simulink model "flexcan_and_fm_over_can_s32k14x"  (Simulink 9.0)
settings: Solver=FixedStepDiscrete  StartTime=0.0  StopTime=10.0  FixedStep=0.1  RelTol=1e-3  EnableMultiTasking=on
InitFcn:
  | mbd_s32k_consistency_checks(bdroot(gcs));
undefined symbols (not defined in the file): LQFP
libraries: mbd_s32k1xx_ec_toolbox x9, simulink x1
Description:
  | This model tests freemaster over CAN0 interface and use CAN1 interface to communicate
  | with other device (eg.: S32K118EVB).
  | 
  | 
  | Validation:
  | 
  | Build flexcan_loopback32k11x.mdl project on S32k118 EVB
  | Build flexcan_and_fm_over_can_s32k14x.mdl on S32k144 EVB
  | Make sure you connect S32K144 through CAN1 interface to S32k118
  | 
  | Open "flexcan_and_fm_over_can_s32k14x.pmp" freemaster project, connect to S32K144
  | board through CAN0 interface at 1Mbps and modify 'CAN_send' variable from Freemaster to '1'.
  | 
  | Once the 'CAN_send' variable is set to 1, a numeric sequence with ID 0x3FF is send once on FlexCAN1 at 500Kbps, Red LED will light
  | for a short period. The S32K144 board will listen for
  | a message with ID 0x3FE over the same CAN1 and once it was received, the 'CAN_send' variable will be cleared.
  | 
  | - The CAN0 (Freemaster) Baudrate is set to 1Mbps and CAN1 Baudrate is set to 500Kbps.
  | -S32K118EVB-Q064 (or any other device who can receive a message over can interface and send back a message with
  | ID 0x3FE)
  | 
  | HW prerequisite:
  | - S32K144EVB-Q100
  | - S32K118EVB-Q064 (or any other device who can receive a message over can interface and send back a message with
  | ID 0x3FE)
  | 
  | - Make sure that external power supply is provided through J16.
settings Model: Creator=agrigorev  LastModifiedBy=nxf35172
settings DataIOCC: ExternalInput=off  InitialState=off  LimitDataPoints=on  SaveOutput=off  SignalLogging=off  SaveTime=off
settings OptimizationCC: DefaultParameterBehavior=Inlined  LifeSpan=1
settings DebuggingCC: SolverPrmCheckMsg=warning  InheritedTsInSrcMsg=none  SingleTaskRateTransMsg=error  UnconnectedInputMsg=error  UnconnectedOutputMsg=error  UnconnectedLineMsg=error  AllowSymbolicDim=off  UnknownTsInhSupMsg=error  StateNameClashWarn=warning
settings HardwareCC: ProdLargestAtomicInteger=Long  ProdLargestAtomicFloat=Double  ProdIntDivRoundTo=Zero  ProdEndianess=LittleEndian  ProdHWDeviceType=ARM Compatible->ARM Cortex
settings SFSimCC: MATLABDynamicMemAlloc=off
settings RTWCC: SystemTargetFile=mbd_s32k.tlc  MakeCommand=mbd_s32k_make_rtw COPY_MDLREF_INCLUDES=0  TemplateMakefile=mbd_s32k.tmf  Description=Model Based Design Toolbox S32K14x Code Generation Target  GenerateReport=on  IncludeHyperlinkInReport=on  LaunchReport=on  GenerateTraceInfo=on  GenerateTraceReport=on  GenerateTraceReportSl=on  GenerateTraceReportSf=on  GenerateTraceReportEml=on
settings CodeAppCC: ForceParamTrailComments=on  IgnoreCustomStorageClasses=off  OperatorAnnotations=on  SimulinkDataObjDesc=on  SFDataObjDesc=on  MATLABFcnDesc=on  InsertBlockDesc=on  MATLABSourceComments=on
settings STFCustomTargetCC: CombineOutputUpdateFcns=on  ERTCustomFileBanners=on  SupportContinuousTime=off  SupportNonInlinedSFcns=off  RemoveResetFunc=on  MATLABClassNameForMDSCustomization=Simulink.SoftwareTarget.ERTCustomization  GRTInterface=off  SystemTargetFile=mbd_s32k14.tlc
settings ERTTargetCC: MultiwordLength=2048  ParMdlRefBuildCompliant=off  CompOptLevelCompliant=off  ConcurrentExecutionCompliant=off  ModelStepFunctionPrototypeControlCompliant=off  CPPClassGenCompliant=off  UseToolchainInfoCompliant=off  InlinedParameterPlacement=NonHierarchical  ERTSrcFileBannerTemplate=mbd_ert_code_template.cgt  ERTHdrFileBannerTemplate=mbd_ert_code_template.cgt  ERTDataSrcFileTemplate=mbd_ert_code_template.cgt  ERTDataHdrFileTemplate=mbd_ert_code_template.cgt  ERTCustomFileTemplate=example_file_process.tlc

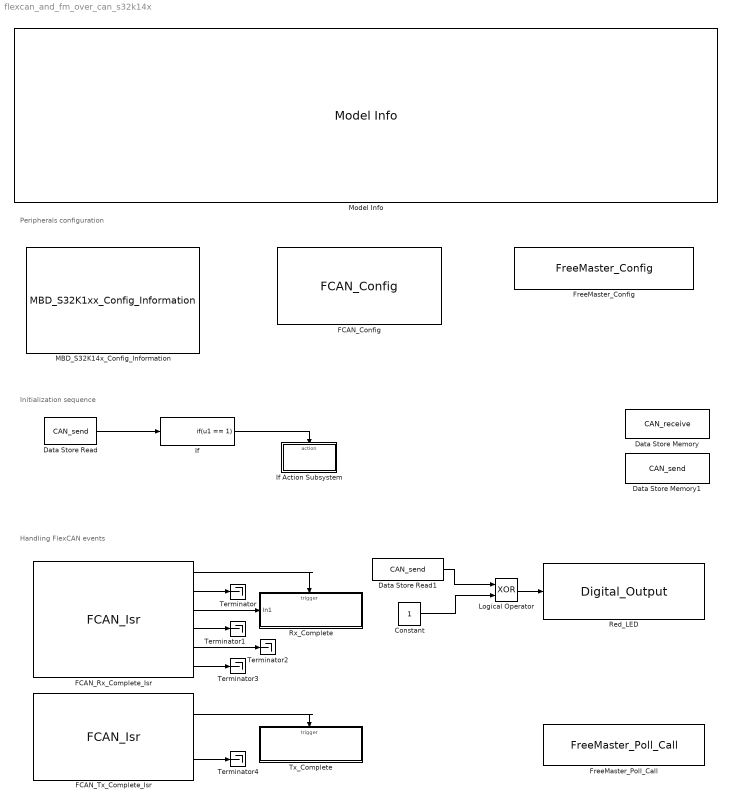
== system flexcan_and_fm_over_can_s32k14x ==
  note: Peripherals configuration
  note: Handling FlexCAN events
  note: Initialization sequence
  Constant : Constant  OutDataTypeStr=boolean
  Data Store Memory : DataStoreMemory  DataStoreName=CAN_receive  ReadBeforeWriteMsg=warning  WriteAfterWriteMsg=warning  WriteAfterReadMsg=warning  ShowAdditionalParam=off  OutDataTypeStr=uint8
  Data Store Memory1 : DataStoreMemory  DataStoreName=CAN_send  ReadBeforeWriteMsg=warning  WriteAfterWriteMsg=warning  WriteAfterReadMsg=warning  ShowAdditionalParam=off  OutDataTypeStr=boolean
  Data Store Read : DataStoreRead  DataStoreName=CAN_send
  Data Store Read1 : DataStoreRead  DataStoreName=CAN_send
  FCAN_Config : mbd_s32k1xx_ec_toolbox/Communication Blocks/CAN Blocks/FCAN_Config  Priority=1  can_instance=1  can_mode=Normal mode  can_max_num_mb=16  can_rx=PTA12: [CAN1_RX | CAN Rx channel]  can_tx=PTA13: [CAN1_TX | CAN Tx Channel]  show_adv_opts=on  can_clk_src=Peripheral clock  bitrate=500  bitrate_adv_opts=off  can_presdiv=7  can_rjw=3  can_pseg1=6  can_pseg2=3  can_propseg=7  can_cbt_presdiv=9  can_cbt_rjw=0  can_cbt_pseg1=3  can_cbt_pseg2=3  can_cbt_propseg=6  can_fd_enable=off  can_payload=8  can_rxfifo_enable=off  can_fifo_id_filter_extended=off  can_fifo_id_filter_remote=off  can_num_id_filters=8  can_fifo_id_format=A  can_fifo_id_filter={'0x0', '0x0', '0x0', '0x0', '0x0', '0x0', '0x0', '0x0'}  can_pn_enable=off  can_wakeup_match=off  can_wakeup_timeout=off  can_timeout_en=off  can_match_timeout=1  can_multiple_matches_en=off  can_num_matches=1  can_idfilter_extendedid=off  can_idfilter_remoteframe=off  can_idfilter_type=Match exact  can_idfilter_id1=0  can_idfilter_id2=0  can_payloadfilter_enable=on  can_payloadfilter_dlclow=0  can_payloadfilter_dlchigh=0  can_payloadfilter_type=Match exact  can_payloadfilter_payload1_b0=0  can_payloadfilter_payload1_b1=0  can_payloadfilter_payload1_b2=0  can_payloadfilter_payload1_b3=0  can_payloadfilter_payload1_b4=0  can_payloadfilter_payload1_b5=0  can_payloadfilter_payload1_b6=0  can_payloadfilter_payload1_b7=0  can_payloadfilter_payload2_b0=0  can_payloadfilter_payload2_b1=0  can_payloadfilter_payload2_b2=0  can_payloadfilter_payload2_b3=0  can_payloadfilter_payload2_b4=0  can_payloadfilter_payload2_b5=0  can_payloadfilter_payload2_b6=0  can_payloadfilter_payload2_b7=0
  FCAN_Rx_Complete_Isr : mbd_s32k1xx_ec_toolbox/Communication Blocks/CAN Blocks/FCAN_Isr  can_instance=1  can_event=Rx Complete
  FCAN_Tx_Complete_Isr : mbd_s32k1xx_ec_toolbox/Communication Blocks/CAN Blocks/FCAN_Isr  can_instance=1  can_event=Tx Complete
  FreeMaster_Config : mbd_s32k1xx_ec_toolbox/Utility Blocks/FreeMaster_Config  interface=CAN0  baudrate=1M  rxd=PTE4: [CAN0_RX | CAN Rx channel]  txd=PTE5: [CAN0_TX | CAN Tx Channel]  mode=Short Interrupt  isr_prio=0  show_adv_opts=on  use_scope=on  max_scope_vars=8  use_recorder=on  max_rec_vars=8  rec_buff_size=512  rec_timebase=10 milliseconds  comm_buffer_size_auto=on  comm_buffer_size=255  comm_rqueue_size_default=on  comm_rqueue_size=32
  FreeMaster_Poll_Call : mbd_s32k1xx_ec_toolbox/Utility Blocks/FreeMaster_Poll_Call
  If : If  IfExpression=u1 == 1  ShowElse=off
  If Action Subsystem : Subsystem  TreatAsAtomicUnit=on
  Logical Operator : Logic  Operator=XOR  AllPortsSameDT=off  OutDataTypeStr=boolean
  MBD_S32K14x_Config_Information : mbd_s32k1xx_ec_toolbox/MBD_S32K1xx_Config_Information  mbdt_ver=0  disp_str=|  config_params=[]  mcu_target_name=S32K144  mcu_target_package=100-LQFP  mcu_target_sram_size=48KB  mcu_system_clock_freq=80  mcu_xtal_freq=External 8  mcu_steptick_timer=LPIT Channel 0  mcu_steptick_prio=15  ds_import_enable=on  target_compiler=GCC  target_memory=FLASH  gcc_target_compile_opts=-mcpu=cortex-m4 -mthumb -mfloat-abi=hard -mfpu=fpv4-sp-d16 -O1 -g -gstrict-dwarf  gcc_target_assemble_opts=-mcpu=cortex-m4 -mthumb -mfloat-abi=hard -mfpu=fpv4-sp-d16 -g  gcc_target_link_opts=-mcpu=cortex-m4 -mthumb -mfloat-abi=hard -mfpu=fpv4-sp-d16  gcc_target_default_lcf=on  gcc_target_user_lcf=S32K144_48_flash.ld  ghs_target_compile_opts=-cpu=cortexm4f -thumb -DARM_MATH_CM4 -fpu=vfpv4_d16 -fsingle -Ogeneral -Wundef -Wimplicit-int -Wshadow -Wtrigraphs --no_commons --gnu_asm -gnu99 -gdwarf-2 -G  ghs_target_assemble_opts=-cpu=cortexm4f -fpu=vfpv4_d16  ghs_target_link_opts=-cpu=cortexm4f -thumb -fpu=vfpv4_d16  ghs_target_default_lcf=on  ghs_target_user_lcf=S32K144_48_flash.ld  iar_target_compile_opts=--cpu=Cortex-M4F --thumb --fpu=VFPv4_sp -Ol -e --debug --dlib_config normal  iar_target_assemble_opts=--cpu Cortex-M4F --thumb --fpu VFPv4_sp  iar_target_link_opts=--no_exceptions --vfe --inline  iar_target_default_lcf=on  iar_target_user_lcf=S32K144_48_flash.icf  pil_download_enable=off  rbl_download_enable=on  rbl_start_delay=5000000  rbl_download_interface=OpenSDA  rbl_restart_request=off  rbl_com_port=Custom  rbl_com_port_custom=COM1  pil_download_rate=57600  pil_opensda_drive=Custom  pil_opensda_drive_custom=D  pil_uart_instance=0  pil_uart_rx=PTA2: [LPUART0_RX | Receive]  pil_uart_tx=PTA3: [LPUART0_TX | Transmit]  FTM_PWM_PcrCheckEnDis=on  FTM_Input_Edge_Inputs_PcrCheckEnDis=on  FTM_Dual_Edge_Inputs_PcrCheckEnDis=on  FTM_Quadrature_Inputs_PcrCheckEnDis=on  FTM_Hall_Sensor_Inputs_PcrCheckEnDis=on  LPTMR_PcrCheckEnDis=on  PIT_PcrCheckEnDis=on  RTC_PcrCheckEnDis=on  FlexCAN_PcrCheckEnDis=on  LIN_PcrCheckEnDis=on  FlexIO_PcrCheckEnDis=on  LPI2C_PcrCheckEnDis=on  LPSPI_PcrCheckEnDis=on  LPUART_PcrCheckEnDis=on  CMP_PcrCheckEnDis=on  GPIO_OutputPcrCheckEnDis=on  GPIO_InputPcrCheckEnDis=on  SBC_PcrCheckEnDis=on  AMMCLIB_PcrCheckEnDis=on  FM_PcrCheckEnDis=on  Profile_PcrCheckEnDis=on  ConfigParams_PcrCheckEnDis=on  ModelRef_PcrCheckEnDis=on  PDB0_PcrCheckEnDis=on  CSEc_PcrCheckEnDis=on  eDMA_PcrCheckEnDis=on  ADC_PcrCheckEnDis=on  WDOG_PcrCheckEnDis=on
      | Target : S32K144-64KB_SRAM
      | Package : 100-pin
      | System clock : 80 MHz
      | XTAL clock : External 8 MHz
      | Compiler : IAR
      | Target Type : FLASH
      | Download Code after build : off
      | Step Tick Interrupt Priority : 15
  Model Info : simulink/Model-Wide Utilities/Model Info  Frame=on  DisplayStringWithTags=|  HorizontalTextAlignment=Left  LeftAlignmentValue=0.02
      | Model Name: %<ModelName>
      | 
      | Description: %<Description>
  Red_LED : mbd_s32k1xx_ec_toolbox/GPIO Blocks/Digital_Output  gpio_pin=PTD15: [PTD15 | Port D I/O]  init_val=Low  drive_strength=Low
  Rx_Complete : Subsystem  TreatAsAtomicUnit=on
      settings: RTWSystemCode=Nonreusable function
  Terminator{,1..4} (5 alike) : Terminator
  Tx_Complete : Subsystem  TreatAsAtomicUnit=on
      settings: RTWSystemCode=Nonreusable function
  wires:
  If/1 -> If Action Subsystem/Action
  Data Store Read/1 -> If/1
  FCAN_Rx_Complete_Isr/1 -> Rx_Complete/Trigger
  FCAN_Rx_Complete_Isr/3 -> Rx_Complete/1(In1)
  FCAN_Tx_Complete_Isr/1 -> Tx_Complete/Trigger
  FCAN_Rx_Complete_Isr/2 -> Terminator/1
  FCAN_Rx_Complete_Isr/4 -> Terminator1/1
  FCAN_Rx_Complete_Isr/5 -> Terminator2/1
  FCAN_Tx_Complete_Isr/2 -> Terminator4/1
  FCAN_Rx_Complete_Isr/6 -> Terminator3/1
  Data Store Read1/1 -> Logical Operator/1
  Logical Operator/1 -> Red_LED/1
  Constant/1 -> Logical Operator/2

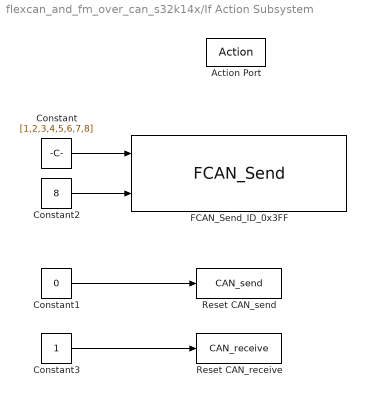
== system flexcan_and_fm_over_can_s32k14x/If Action Subsystem ==
  Action Port : ActionPort  ActionType=then
  Constant : Constant  Value=[1,2,3,4,5,6,7,8]  OutDataTypeStr=uint8
  Constant1 : Constant  Value=0  OutDataTypeStr=boolean
  Constant2 : Constant  Value=8  OutDataTypeStr=uint8
  Constant3 : Constant  OutDataTypeStr=uint8
  FCAN_Send_ID_0x3FF : mbd_s32k1xx_ec_toolbox/Communication Blocks/CAN Blocks/FCAN_Send  Priority=2  can_instance=1  can_mode=Non-blocking  can_timeout_ms=0  can_mb_idx=15  can_extended_id=off  can_is_remote=off  can_id=3FF  show_adv_opts=off  can_fd_enable=off  can_enable_brs=off  can_fd_padding=0
  Reset CAN_receive : DataStoreWrite  DataStoreName=CAN_receive
  Reset CAN_send : DataStoreWrite  DataStoreName=CAN_send
  wires:
  Constant/1 -> FCAN_Send_ID_0x3FF/1
  Constant2/1 -> FCAN_Send_ID_0x3FF/2
  Constant1/1 -> Reset CAN_send/1
  Constant3/1 -> Reset CAN_receive/1

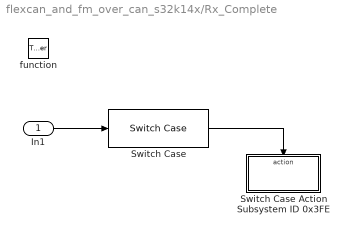
== system flexcan_and_fm_over_can_s32k14x/Rx_Complete ==
  In1 : Inport
  function : TriggerPort  TriggerType=function-call  VariantControl=Variant
  Switch Case : SwitchCase  CaseConditions={hex2dec('3FE')}  ShowDefaultCase=off
  Switch Case Action Subsystem ID 0x3FE : Subsystem  TreatAsAtomicUnit=on
  wires:
  In1/1 -> Switch Case/1
  Switch Case/1 -> Switch Case Action Subsystem ID 0x3FE/Action

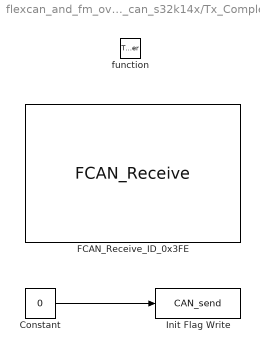
== system flexcan_and_fm_over_can_s32k14x/Tx_Complete ==
  function : TriggerPort  TriggerType=function-call  VariantControl=Variant
  Constant : Constant  Value=0  OutDataTypeStr=boolean
  FCAN_Receive_ID_0x3FE : mbd_s32k1xx_ec_toolbox/Communication Blocks/CAN Blocks/FCAN_Receive  can_instance=1  can_mode=Non-blocking  can_timeout_ms=0  can_mb_idx=14  can_extended_id=off  can_is_remote=off  can_id=3FE  can_msg_mask=FFFFFFFF  show_adv_opts=off  can_use_rxfifo=off  can_fd_enable=off
  Init Flag Write : DataStoreWrite  DataStoreName=CAN_send
  wires:
  Constant/1 -> Init Flag Write/1

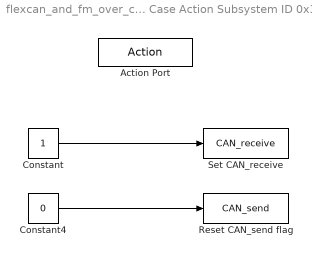
== system flexcan_and_fm_over_can_s32k14x/Rx_Complete/Switch Case Action Subsystem ID 0x3FE ==
  Action Port : ActionPort  ActionType=case
  Constant : Constant  OutDataTypeStr=uint8
  Constant4 : Constant  Value=0  OutDataTypeStr=boolean
  Reset CAN_send flag : DataStoreWrite  DataStoreName=CAN_send
  Set CAN_receive : DataStoreWrite  DataStoreName=CAN_receive
  wires:
  Constant/1 -> Set CAN_receive/1
  Constant4/1 -> Reset CAN_send flag/1
